simulink library "halout"  (R2021b)
settings: Solver=VariableStepAuto  StartTime=0.0  StopTime=10.0  RelTol=1e-3
undefined symbols (not defined in the file): C_TASK_5MS_S, FALSE, KHAL_CAN1FD1APS3E2E_flg, KHAL_CAN1FD1APS3TxReq_flg, KHAL_CAN1FD1VCU2E2E_flg, KHAL_CAN1FD1VCU2TxReq_flg, KHAL_CAN1FD1VCU3E2E_flg, KHAL_CAN1FD1VCU3TxReq_flg, KHAL_CAN1TxReq_flg, KHAL_CAN1VMCFCM1E2E_flg, KHAL_CAN1VMCFCM1TxReq_flg, KHAL_CAN2TxReq_flg, KHAL_CAN3FD3VCU1toNIDECTxReq_flg, KHAL_CAN3FD3VCU1TxReq_flg, KHAL_CAN3FD3VCU2E2E_flg, KHAL_CAN3FD3VCU2toNIDECE2E_flg, KHAL_CAN3FD3VCU2toNIDECTxReq_flg, KHAL_CAN3FD3VCU2TxReq_flg, KHAL_CAN3TxReq_flg, KHAL_CAN4FD4CE1000E2E_flg, KHAL_CAN4FD4CE1000TxReq_flg, KHAL_CAN4TxReq_flg, KHAL_CAN5TxReq_flg, KHAL_CAN6FD6APS3E2E_flg, KHAL_CAN6FD6APS3TxReq_flg, KHAL_CAN6FD6VCU2E2E_flg, KHAL_CAN6FD6VCU2TxReq_flg, KHAL_CAN6TxReq_flg, ONE_INT, TRUE, ZERO_INT
libraries: FVT_lib x549, simulink x244
(part 3 of 27)

== system halout/HAL_OUT/CAN1/FD1_VCU1_0x116 ==
  BSCP_outputs : Inport  OutDataTypeStr=Bus: BSCP_outputs
  BOUTP_outputs : Inport  Port=2  OutDataTypeStr=Bus: BOUTP_outputs
  CCCrlSta : Subsystem
  EngAGSCloseSta : Subsystem
  EngActvDmpDisabSta : Subsystem
  EngCoastDwSta : Subsystem
  EngPwrLockSta : Subsystem
  Ground{,1..3} (4 alike) : Ground
  HVPwrSta : Subsystem
  LVPwrSta : Subsystem
  MSACrlSta : Subsystem
  PButtonSta : Subsystem
  PrkReq : Subsystem
  PrkReqValid : Subsystem
  PwrSta : Subsystem
  ShiftGearPosn : Subsystem
  VehMalfunLevel : Subsystem
  XWDMode : Subsystem
  bus_creator : BusCreator  Inputs=15  OutDataTypeStr=Bus: DT_CAN1_SG_FD1_VCU1  NonVirtualBus=on
  bus_selector : BusSelector  OutputSignals=VOUTP_CCCtrlSta_enum
  bus_selector1 : BusSelector  OutputSignals=VOUTP_IVIPwrLockSta_enum
  bus_selector10 : BusSelector  OutputSignals=VOUTP_DrivetrainSelect_enum
  bus_selector2 : BusSelector  OutputSignals=VOUTP_HVPwrSta_flg
  bus_selector3 : BusSelector  OutputSignals=VOUTP_LVPwrSta_flg
  bus_selector4 : BusSelector  OutputSignals=VOUTP_MSACtrlSta_enum
  bus_selector5 : BusSelector  OutputSignals=VOUTP_PButtonSta_enum
  bus_selector6 : BusSelector  OutputSignals=VOUTP_ActParkRequest_flg
  bus_selector7 : BusSelector  OutputSignals=VOUTP_PowerSta_enum
  bus_selector8 : BusSelector  OutputSignals=VOUTP_ShiftGearPosn_enum
  bus_selector9 : BusSelector  OutputSignals=VOUTP_VehMalfunLevel_enum
  FD1_VCU1 : Outport
  wires:
  BSCP_outputs/1 -> [BSCP_outputs]
  BOUTP_outputs/1 -> [BOUTP_outputs]
  [CAN1_CC_Crl_Sta] -> bus_creator/1  "CAN1_CC_Crl_Sta"
  [CAN1_Eng_AGSCloseSta] -> bus_creator/2  "CAN1_Eng_AGSCloseSta"
  [CAN1_Eng_ActvDmpDisabSta] -> bus_creator/3  "CAN1_Eng_ActvDmpDisabSta"
  [CAN1_Eng_CoastDwSta] -> bus_creator/4  "CAN1_Eng_CoastDwSta"
  [CAN1_Eng_PwrLockSta] -> bus_creator/5  "CAN1_Eng_PwrLockSta"
  [CAN1_HVPwrSta] -> bus_creator/6  "CAN1_HVPwrSta"
  [CAN1_LVPwrSta] -> bus_creator/7  "CAN1_LVPwrSta"
  [CAN1_MSA_Crl_Sta] -> bus_creator/8  "CAN1_MSA_Crl_Sta"
  [CAN1_P_Button_Sta] -> bus_creator/9  "CAN1_P_Button_Sta"
  [CAN1_PrkReq] -> bus_creator/10  "CAN1_PrkReq"
  [CAN1_PrkReqValid] -> bus_creator/11  "CAN1_PrkReqValid"
  [CAN1_PwrSta] -> bus_creator/12  "CAN1_PwrSta"
  [CAN1_ShiftGearPosn] -> bus_creator/13  "CAN1_ShiftGearPosn"
  [CAN1_VehMalfunLevel] -> bus_creator/14  "CAN1_VehMalfunLevel"
  [CAN1_XWDMode] -> bus_creator/15  "CAN1_XWDMode"
  bus_creator/1 -> FD1_VCU1/1
  CCCrlSta/1(CAN1_CC_Crl_Sta) -> [CAN1_CC_Crl_Sta]
  EngAGSCloseSta/1(CAN1_Eng_AGSCloseSta) -> [CAN1_Eng_AGSCloseSta]
  EngActvDmpDisabSta/1(CAN1_Eng_ActvDmpDisabSta) -> [CAN1_Eng_ActvDmpDisabSta]
  EngCoastDwSta/1(CAN1_Eng_CoastDwSta) -> [CAN1_Eng_CoastDwSta]
  EngPwrLockSta/1(CAN1_Eng_PwrLockSta) -> [CAN1_Eng_PwrLockSta]
  HVPwrSta/1(CAN1_HVPwrSta) -> [CAN1_HVPwrSta]
  LVPwrSta/1(CAN1_LVPwrSta) -> [CAN1_LVPwrSta]
  MSACrlSta/1(CAN1_MSA_Crl_Sta) -> [CAN1_MSA_Crl_Sta]
  PButtonSta/1(CAN1_P_Button_Sta) -> [CAN1_P_Button_Sta]
  PrkReq/1(CAN1_PrkReq) -> [CAN1_PrkReq]
  PrkReqValid/1(CAN1_PrkReqValid) -> [CAN1_PrkReqValid]
  PwrSta/1(CAN1_PwrSta) -> [CAN1_PwrSta]
  ShiftGearPosn/1(CAN1_ShiftGearPosn) -> [CAN1_ShiftGearPosn]
  VehMalfunLevel/1(CAN1_VehMalfunLevel) -> [CAN1_VehMalfunLevel]
  XWDMode/1(CAN1_XWDMode) -> [CAN1_XWDMode]
  bus_selector/1 -> CCCrlSta/1(CCCrlSta)  "<VOUTP_CCCtrlSta_enum>"
  [BOUTP_outputs] -> bus_selector/1
  Ground/1 -> EngAGSCloseSta/1(EngAGSCloseSta)
  Ground1/1 -> EngActvDmpDisabSta/1(EngActvDmpDisabSta)
  Ground2/1 -> EngCoastDwSta/1(EngCoastDwSta)
  bus_selector1/1 -> EngPwrLockSta/1(EngPwrLockSta)  "<VOUTP_IVIPwrLockSta_enum>"
  [BOUTP_outputs] -> bus_selector1/1
  bus_selector2/1 -> HVPwrSta/1(HVPwrSta)  "<VOUTP_HVPwrSta_flg>"
  [BOUTP_outputs] -> bus_selector2/1
  bus_selector3/1 -> LVPwrSta/1(LVPwrSta)  "<VOUTP_LVPwrSta_flg>"
  [BOUTP_outputs] -> bus_selector3/1
  bus_selector4/1 -> MSACrlSta/1(MSACrlSta)  "<VOUTP_MSACtrlSta_enum>"
  [BOUTP_outputs] -> bus_selector4/1
  bus_selector5/1 -> PButtonSta/1(PButtonSta)  "<VOUTP_PButtonSta_enum>"
  [BOUTP_outputs] -> bus_selector5/1
  bus_selector6/1 -> PrkReq/1(PrkReq)  "<VOUTP_ActParkRequest_flg>"
  [BOUTP_outputs] -> bus_selector6/1
  Ground3/1 -> PrkReqValid/1(PrkReqValid)
  bus_selector7/1 -> PwrSta/1(PwrSta)  "<VOUTP_PowerSta_enum>"
  [BOUTP_outputs] -> bus_selector7/1
  bus_selector8/1 -> ShiftGearPosn/1(ShiftGearPosn)  "<VOUTP_ShiftGearPosn_enum>"
  [BOUTP_outputs] -> bus_selector8/1
  bus_selector9/1 -> VehMalfunLevel/1(VehMalfunLevel)  "<VOUTP_VehMalfunLevel_enum>"
  [BOUTP_outputs] -> bus_selector9/1
  bus_selector10/1 -> XWDMode/1(XWDMode)  "<VOUTP_DrivetrainSelect_enum>"
  [BOUTP_outputs] -> bus_selector10/1

== system halout/HAL_OUT/CAN1/FD1_VCU2_0x154 ==
  BSCP_outputs : Inport  OutDataTypeStr=Bus: BSCP_outputs
  BOUTP_outputs : Inport  Port=2  OutDataTypeStr=Bus: BOUTP_outputs
  Trigger : TriggerPort  TriggerType=function-call  VariantControl=(inherit)
  ACCCtrlAvail : Subsystem
  AccPedalOverride : Subsystem
  ActAPSPosn : Subsystem
  Byte_0 : Subsystem
  Byte_1 : Subsystem
  Byte_10 : Subsystem
  Byte_11 : Subsystem
  Byte_12 : Subsystem
  Byte_13 : Subsystem
  Byte_14 : Subsystem
  Byte_15 : Subsystem
  Byte_2 : Subsystem
  Byte_3 : Subsystem
  Byte_4 : Subsystem
  Byte_5 : Subsystem
  Byte_6 : Subsystem
  Byte_7 : Constant  Value=ZERO_INT
  Byte_8 : Constant  Value=ZERO_INT
  Byte_9 : Constant  Value=ZERO_INT
  CRC8_IfAction_Tx : Subsystem  AncestorBlock=FVT_lib/hal/CRC8_IfAction_Tx
      mask help: MeasumentTrigerEvent
      mask Display: fprintf('CRC8_IfAction');
  CSVCU2CAN1 : Subsystem
  Constant : Constant  Value=KHAL_CAN1FD1VCU2E2E_flg
  Constant1 : Constant  Value=0x2D
  Constant2 : Constant  Value=0xA6
  Constant3 : Constant  Value=KHAL_CAN1FD1VCU2E2E_flg
  Constant4 : Constant  Value=KHAL_CAN1FD1VCU2E2E_flg
  DriverTq : Subsystem
  FrDriverTq : Subsystem
  Ground{,1..7} (8 alike) : Ground
  Mux2 : Mux  Inputs=15
  RCVCU2CAN1 : Subsystem
  RollingCounter_IfAction : FVT_lib/hal/RollingCounter_IfAction
  RollingCounter_IfAction1 : FVT_lib/hal/RollingCounter_IfAction
  RrDriverTq : Subsystem
  Terminator : Terminator
  VehActPwr : Subsystem
  bus_creator : BusCreator  Inputs=9  OutDataTypeStr=Bus: DT_CAN1_SG_FD1_VCU2  NonVirtualBus=on
  bus_selector : BusSelector  OutputSignals=VOUTP_DriverWhlTqDemFr_Nm
  bus_selector1 : BusSelector  OutputSignals=VOUTP_DriverWhlTqDemFr_Nm
  bus_selector10 : BusSelector  OutputSignals=VOUTP_DriverWhlTqDemFr_Nm
  bus_selector11 : BusSelector  OutputSignals=VOUTP_DriverWhlTqDemRr_Nm
  bus_selector2 : BusSelector  OutputSignals=VOUTP_DriverWhlTqDemRr_Nm
  bus_selector3 : BusSelector  OutputSignals=VOUTP_DriverWhlTqDemRr_Nm
  bus_selector4 : BusSelector  OutputSignals=VOUTP_ACCCtrlAvail_flg
  bus_selector5 : BusSelector  OutputSignals=VOUTP_ACCPedalOvrd_flg
  bus_selector6 : BusSelector  OutputSignals=VOUTP_ActAPSPosn_pct
  bus_selector7 : BusSelector  OutputSignals=VOUTP_ACCCtrlAvail_flg
  bus_selector8 : BusSelector  OutputSignals=VOUTP_ACCPedalOvrd_flg
  bus_selector9 : BusSelector  OutputSignals=VOUTP_ActAPSPosn_pct
  FD1_VCU2 : Outport
  wires:
  BSCP_outputs/1 -> [BSCP_outputs]
  BOUTP_outputs/1 -> [BOUTP_outputs]
  [CAN1_ACC_CtrlAvail] -> bus_creator/1  "CAN1_ACC_CtrlAvail"
  [CAN1_AccPedal_Override] -> bus_creator/2  "CAN1_AccPedal_Override"
  [CAN1_ActAPSPosn] -> bus_creator/3  "CAN1_ActAPSPosn"
  [CAN1_CS_VCU2_CAN1] -> bus_creator/4  "CAN1_CS_VCU2_CAN1"
  [CAN1_DriverTq] -> bus_creator/5  "CAN1_DriverTq"
  [CAN1_Fr_DriverTq] -> bus_creator/6  "CAN1_Fr_DriverTq"
  [CAN1_RC_VCU2_CAN1] -> bus_creator/7  "CAN1_RC_VCU2_CAN1"
  [CAN1_Rr_DriverTq] -> bus_creator/8  "CAN1_Rr_DriverTq"
  [CAN1_VehActPwr] -> bus_creator/9  "CAN1_VehActPwr"
  bus_creator/1 -> FD1_VCU2/1
  ACCCtrlAvail/1(CAN1_ACC_CtrlAvail) -> [CAN1_ACC_CtrlAvail]
  AccPedalOverride/1(CAN1_AccPedal_Override) -> [CAN1_AccPedal_Override]
  ActAPSPosn/1(CAN1_ActAPSPosn) -> [CAN1_ActAPSPosn]
  CSVCU2CAN1/1(CAN1_CS_VCU2_CAN1) -> [CAN1_CS_VCU2_CAN1]
  DriverTq/1(CAN1_DriverTq) -> [CAN1_DriverTq]
  FrDriverTq/1(CAN1_Fr_DriverTq) -> [CAN1_Fr_DriverTq]
  RCVCU2CAN1/1(CAN1_RC_VCU2_CAN1) -> [CAN1_RC_VCU2_CAN1]
  RrDriverTq/1(CAN1_Rr_DriverTq) -> [CAN1_Rr_DriverTq]
  VehActPwr/1(CAN1_VehActPwr) -> [CAN1_VehActPwr]
  Byte_0/1(Byte_0) -> Terminator/1
  Byte_1/1(Byte_1) -> [Byte_1]
  Byte_2/1(Byte_2) -> [Byte_2]
  Byte_3/1(Byte_3) -> [Byte_3]
  Byte_4/1(Byte_4) -> [Byte_4]
  Byte_5/1(Byte_5) -> [Byte_5]
  Byte_6/1(Byte_6) -> [Byte_6]
  Byte_7/1 -> [Byte_7]
  Byte_8/1 -> [Byte_8]
  Byte_9/1 -> [Byte_9]
  Byte_10/1(Byte_10) -> [Byte_10]
  Byte_11/1(Byte_11) -> [Byte_11]
  Byte_12/1(Byte_12) -> [Byte_12]
  Byte_13/1(Byte_13) -> [Byte_13]
  Byte_14/1(Byte_14) -> [Byte_14]
  Byte_15/1(Byte_15) -> [Byte_15]
  Mux2/1 -> CRC8_IfAction_Tx/4(RawData)
  Constant/1 -> CRC8_IfAction_Tx/1(CAN_E2E_flg)
  Constant1/1 -> CRC8_IfAction_Tx/2(DataID1)
  Constant2/1 -> CRC8_IfAction_Tx/3(DataID2)
  CRC8_IfAction_Tx/1(CRC8) -> [CS_VCU2_CAN1]
  Ground/1 -> Byte_0/1(CS_VCU2_CAN1)
  [Byte_1] -> Mux2/1
  RollingCounter_IfAction/1 -> Byte_1/1(RC_VCU2_CAN1)
  Constant3/1 -> RollingCounter_IfAction/1
  [Byte_2] -> Mux2/2
  bus_selector/1 -> Byte_2/1(Fr_DriverTq)  "<VOUTP_DriverWhlTqDemFr_Nm>"
  [BOUTP_outputs] -> bus_selector/1
  [Byte_3] -> Mux2/3
  bus_selector1/1 -> Byte_3/1(Fr_DriverTq)  "<VOUTP_DriverWhlTqDemFr_Nm>"
  [BOUTP_outputs] -> bus_selector1/1
  [Byte_4] -> Mux2/4
  bus_selector2/1 -> Byte_4/1(Rr_DriverTq)  "<VOUTP_DriverWhlTqDemRr_Nm>"
  [BOUTP_outputs] -> bus_selector2/1
  [Byte_5] -> Mux2/5
  bus_selector3/1 -> Byte_5/1(Rr_DriverTq)  "<VOUTP_DriverWhlTqDemRr_Nm>"
  [BOUTP_outputs] -> bus_selector3/1
  [Byte_6] -> Mux2/6
  bus_selector4/1 -> Byte_6/1(ACC_CtrlAvail)  "<VOUTP_ACCCtrlAvail_flg>"
  [BOUTP_outputs] -> bus_selector4/1
  bus_selector5/1 -> Byte_6/2(AccPedal_Override)  "<VOUTP_ACCPedalOvrd_flg>"
  [BOUTP_outputs] -> bus_selector5/1
  [Byte_7] -> Mux2/7
  [Byte_8] -> Mux2/8
  [Byte_9] -> Mux2/9
  [Byte_10] -> Mux2/10
  Ground1/1 -> Byte_10/1(VehActPwr)
  [Byte_11] -> Mux2/11
  Ground2/1 -> Byte_11/1(VehActPwr)
  [Byte_12] -> Mux2/12
  Ground3/1 -> Byte_12/1(VehActPwr)
  [Byte_13] -> Mux2/13
  Ground4/1 -> Byte_13/1(DriverTq)
  [Byte_14] -> Mux2/14
  Ground5/1 -> Byte_14/1(DriverTq)
  [Byte_15] -> Mux2/15
  bus_selector6/1 -> Byte_15/1(ActAPSPosn)  "<VOUTP_ActAPSPosn_pct>"
  [BOUTP_outputs] -> bus_selector6/1
  bus_selector7/1 -> ACCCtrlAvail/1(ACCCtrlAvail)  "<VOUTP_ACCCtrlAvail_flg>"
  [BOUTP_outputs] -> bus_selector7/1
  bus_selector8/1 -> AccPedalOverride/1(AccPedalOverride)  "<VOUTP_ACCPedalOvrd_flg>"
  [BOUTP_outputs] -> bus_selector8/1
  bus_selector9/1 -> ActAPSPosn/1(ActAPSPosn)  "<VOUTP_ActAPSPosn_pct>"
  [BOUTP_outputs] -> bus_selector9/1
  [CS_VCU2_CAN1] -> CSVCU2CAN1/1(CSVCU2CAN1)
  Ground6/1 -> DriverTq/1(DriverTq)
  bus_selector10/1 -> FrDriverTq/1(FrDriverTq)  "<VOUTP_DriverWhlTqDemFr_Nm>"
  [BOUTP_outputs] -> bus_selector10/1
  RollingCounter_IfAction1/1 -> RCVCU2CAN1/1(RCVCU2CAN1)
  Constant4/1 -> RollingCounter_IfAction1/1
  bus_selector11/1 -> RrDriverTq/1(RrDriverTq)  "<VOUTP_DriverWhlTqDemRr_Nm>"
  [BOUTP_outputs] -> bus_selector11/1
  Ground7/1 -> VehActPwr/1(VehActPwr)

== system halout/HAL_OUT/CAN1/FD1_VCU2_Tx ==
  TxReq : Inport
  Chart : Stateflow chart  TreatAsAtomicUnit=on
  Constant : Constant  Value=C_TASK_5MS_S
  Constant3 : Constant  Value=CycleTime
  Data Type Conversion : DataTypeConversion  OutDataTypeStr=uint16
  Divide : Product  Inputs=*/
  Gain : Gain  Gain=0.001
  TxTrigger : Outport
  wires:
  Data Type Conversion/1 -> Chart/2(CycleCnt)
  Constant3/1 -> Gain/1
  Gain/1 -> Divide/1
  Chart/1(TxTrigger()) -> TxTrigger/1
  Divide/1 -> Data Type Conversion/1
  TxReq/1 -> Chart/1(TxReq)
  Constant/1 -> Divide/2

== system halout/HAL_OUT/CAN1/FD1_VCU3_0x159 ==
  BSCP_outputs : Inport  OutDataTypeStr=Bus: BSCP_outputs
  BOUTP_outputs : Inport  Port=2  OutDataTypeStr=Bus: BOUTP_outputs
  Trigger : TriggerPort  TriggerType=function-call  VariantControl=(inherit)
  Byte_0 : Subsystem
  Byte_1 : Subsystem
  Byte_10 : Subsystem
  Byte_11 : Subsystem
  Byte_12 : Subsystem
  Byte_13 : Subsystem
  Byte_14 : Subsystem
  Byte_15 : Subsystem
  Byte_16 : Subsystem
  Byte_17 : Subsystem
  Byte_18 : Subsystem
  Byte_19 : Subsystem
  Byte_2 : Constant  Value=ZERO_INT
  Byte_3 : Subsystem
  Byte_4 : Subsystem
  Byte_5 : Subsystem
  Byte_6 : Subsystem
  Byte_7 : Subsystem
  Byte_8 : Subsystem
  Byte_9 : Subsystem
  CRC8_IfAction_Tx : Subsystem  AncestorBlock=FVT_lib/hal/CRC8_IfAction_Tx
      mask help: MeasumentTrigerEvent
      mask Display: fprintf('CRC8_IfAction');
  CSVCU3CAN1 : Subsystem
  Constant : Constant  Value=KHAL_CAN1FD1VCU3E2E_flg
  Constant1 : Constant  Value=0xC8
  Constant2 : Constant  Value=0xEB
  Constant3 : Constant  Value=KHAL_CAN1FD1VCU3E2E_flg
  Constant4 : Constant  Value=KHAL_CAN1FD1VCU3E2E_flg
  EquivAccPedalSWSta : Subsystem
  FrEDUAvailBrkRgnTq : Subsystem
  FrEDUAvailBrkRgnTqValid : Subsystem
  FrEDURealARgnTq : Subsystem
  FrEDURealDrvOrBRgnTq : Subsystem
  FrEDUSpd : Subsystem
  FrEDUSpdValid : Subsystem
  FrRgnDecrSta : Subsystem
  FrRgnPermSta : Subsystem
  Ground : Ground
  Mux2 : Mux  Inputs=19
  PTCSPermSta : Subsystem
  RCVCU3CAN1 : Subsystem
  RgnAbnorSta : Subsystem
  RollingCounter_IfAction : FVT_lib/hal/RollingCounter_IfAction
  RollingCounter_IfAction1 : FVT_lib/hal/RollingCounter_IfAction
  RrEDUAvailBrkRgnTq : Subsystem
  RrEDUAvailBrkRgnTqValid : Subsystem
  RrEDURealARgnTq : Subsystem
  RrEDURealDrvOrBRgnTq : Subsystem
  RrEDUSpd : Subsystem
  RrEDUSpdValid : Subsystem
  RrRgnDecrSta : Subsystem
  RrRgnPermSta : Subsystem
  Terminator : Terminator
  bus_creator : BusCreator  Inputs=21  OutDataTypeStr=Bus: DT_CAN1_SG_FD1_VCU3  NonVirtualBus=on
  bus_selector : BusSelector  OutputSignals=VOUTP_FrEDUSpdValid_flg
  bus_selector1 : BusSelector  OutputSignals=VOUTP_FrRgnDecrSta_flg
  bus_selector10 : BusSelector  OutputSignals=VOUTP_RrEDUSpd_rpm
  bus_selector11 : BusSelector  OutputSignals=VOUTP_RrEDURolRgnTq_Nm
  bus_selector12 : BusSelector  OutputSignals=VOUTP_RrEDURolRgnTq_Nm
  bus_selector13 : BusSelector  OutputSignals=VOUTP_RrEDUAvailBrkRgnTq_Nm
  bus_selector14 : BusSelector  OutputSignals=VOUTP_RrEDUAvailBrkRgnTq_Nm
  bus_selector15 : BusSelector  OutputSignals=VOUTP_RrEDUActTq_Nm
  bus_selector16 : BusSelector  OutputSignals=VOUTP_RrEDUActTq_Nm
  bus_selector17 : BusSelector  OutputSignals=VOUTP_FrEDUAvailBrkRgnTqV_flg
  bus_selector18 : BusSelector  OutputSignals=VOUTP_FrEDUSpd_rpm
  bus_selector19 : BusSelector  OutputSignals=VOUTP_RrEDUAvailBrkRgnTqV_flg
  bus_selector2 : BusSelector  OutputSignals=VOUTP_FrRgnPermSta_flg
  bus_selector20 : BusSelector  OutputSignals=VOUTP_FrEDUSpd_rpm
  bus_selector21 : BusSelector  OutputSignals=VOUTP_FrEDURolRgnTq_Nm
  bus_selector22 : BusSelector  OutputSignals=VOUTP_FrEDURolRgnTq_Nm
  bus_selector23 : BusSelector  OutputSignals=VOUTP_FrEDUAvailBrkRgnTq_Nm
  bus_selector24 : BusSelector  OutputSignals=VOUTP_FrEDUAvailBrkRgnTq_Nm
  bus_selector25 : BusSelector  OutputSignals=VOUTP_FrEDUActTq_Nm
  bus_selector26 : BusSelector  OutputSignals=VOUTP_FrEDUActTq_Nm
  bus_selector27 : BusSelector  OutputSignals=VOUTP_EquivAccPedalSWSta_flg
  bus_selector28 : BusSelector  OutputSignals=VOUTP_FrEDUAvailBrkRgnTq_Nm
  bus_selector29 : BusSelector  OutputSignals=VOUTP_FrEDUAvailBrkRgnTqV_flg
  bus_selector3 : BusSelector  OutputSignals=VOUTP_RgnAbnorSta_flg
  bus_selector30 : BusSelector  OutputSignals=VOUTP_FrEDURolRgnTq_Nm
  bus_selector31 : BusSelector  OutputSignals=VOUTP_FrEDUActTq_Nm
  bus_selector32 : BusSelector  OutputSignals=VOUTP_FrEDUSpd_rpm
  bus_selector33 : BusSelector  OutputSignals=VOUTP_FrEDUSpdValid_flg
  bus_selector34 : BusSelector  OutputSignals=VOUTP_FrRgnDecrSta_flg
  bus_selector35 : BusSelector  OutputSignals=VOUTP_FrRgnPermSta_flg
  bus_selector36 : BusSelector  OutputSignals=VOUTP_PTCSPermSta_flg
  bus_selector37 : BusSelector  OutputSignals=VOUTP_RgnAbnorSta_flg
  bus_selector38 : BusSelector  OutputSignals=VOUTP_RrEDUAvailBrkRgnTq_Nm
  bus_selector39 : BusSelector  OutputSignals=VOUTP_RrEDUAvailBrkRgnTqV_flg
  bus_selector4 : BusSelector  OutputSignals=VOUTP_RrEDUSpdValid_flg
  bus_selector40 : BusSelector  OutputSignals=VOUTP_RrEDURolRgnTq_Nm
  bus_selector41 : BusSelector  OutputSignals=VOUTP_RrEDUActTq_Nm
  bus_selector42 : BusSelector  OutputSignals=VOUTP_RrEDUSpd_rpm
  bus_selector43 : BusSelector  OutputSignals=VOUTP_RrEDUSpdValid_flg
  bus_selector44 : BusSelector  OutputSignals=VOUTP_RrRgnDecrSta_flg
  bus_selector45 : BusSelector  OutputSignals=VOUTP_RrRgnPermSta_flg
  bus_selector5 : BusSelector  OutputSignals=VOUTP_RrRgnDecrSta_flg
  bus_selector6 : BusSelector  OutputSignals=VOUTP_RrRgnPermSta_flg
  bus_selector7 : BusSelector  OutputSignals=VOUTP_EquivAccPedalSWSta_flg
  bus_selector8 : BusSelector  OutputSignals=VOUTP_PTCSPermSta_flg
  bus_selector9 : BusSelector  OutputSignals=VOUTP_RrEDUSpd_rpm
  FD1_VCU3 : Outport
  wires:
  BSCP_outputs/1 -> [BSCP_outputs]
  BOUTP_outputs/1 -> [BOUTP_outputs]
  [CAN1_CS_VCU3_CAN1] -> bus_creator/1  "CAN1_CS_VCU3_CAN1"
  [CAN1_EquivAccPedalSWSta] -> bus_creator/2  "CAN1_EquivAccPedalSWSta"
  [CAN1_Fr_EDUAvailBrkRgnTq] -> bus_creator/3  "CAN1_Fr_EDUAvailBrkRgnTq"
  [CAN1_Fr_EDUAvailBrkRgnTqValid] -> bus_creator/4  "CAN1_Fr_EDUAvailBrkRgnTqValid"
  [CAN1_Fr_EDURealARgnTq] -> bus_creator/5  "CAN1_Fr_EDURealARgnTq"
  [CAN1_Fr_EDURealDrvOrBRgnTq] -> bus_creator/6  "CAN1_Fr_EDURealDrvOrBRgnTq"
  [CAN1_Fr_EDUSpd] -> bus_creator/7  "CAN1_Fr_EDUSpd"
  [CAN1_Fr_EDUSpdValid] -> bus_creator/8  "CAN1_Fr_EDUSpdValid"
  [CAN1_Fr_RgnDecrSta] -> bus_creator/9  "CAN1_Fr_RgnDecrSta"
  [CAN1_Fr_RgnPermSta] -> bus_creator/10  "CAN1_Fr_RgnPermSta"
  [CAN1_PTCS_PermSta] -> bus_creator/11  "CAN1_PTCS_PermSta"
  [CAN1_RC_VCU3_CAN1] -> bus_creator/12  "CAN1_RC_VCU3_CAN1"
  [CAN1_RgnAbnorSta] -> bus_creator/13  "CAN1_RgnAbnorSta"
  [CAN1_Rr_EDUAvailBrkRgnTq] -> bus_creator/14  "CAN1_Rr_EDUAvailBrkRgnTq"
  [CAN1_Rr_EDUAvailBrkRgnTqValid] -> bus_creator/15  "CAN1_Rr_EDUAvailBrkRgnTqValid"
  [CAN1_Rr_EDURealARgnTq] -> bus_creator/16  "CAN1_Rr_EDURealARgnTq"
  [CAN1_Rr_EDURealDrvOrBRgnTq] -> bus_creator/17  "CAN1_Rr_EDURealDrvOrBRgnTq"
  [CAN1_Rr_EDUSpd] -> bus_creator/18  "CAN1_Rr_EDUSpd"
  [CAN1_Rr_EDUSpdValid] -> bus_creator/19  "CAN1_Rr_EDUSpdValid"
  [CAN1_Rr_RgnDecrSta] -> bus_creator/20  "CAN1_Rr_RgnDecrSta"
  [CAN1_Rr_RgnPermSta] -> bus_creator/21  "CAN1_Rr_RgnPermSta"
  bus_creator/1 -> FD1_VCU3/1
  CSVCU3CAN1/1(CAN1_CS_VCU3_CAN1) -> [CAN1_CS_VCU3_CAN1]
  EquivAccPedalSWSta/1(CAN1_EquivAccPedalSWSta) -> [CAN1_EquivAccPedalSWSta]
  FrEDUAvailBrkRgnTq/1(CAN1_Fr_EDUAvailBrkRgnTq) -> [CAN1_Fr_EDUAvailBrkRgnTq]
  FrEDUAvailBrkRgnTqValid/1(CAN1_Fr_EDUAvailBrkRgnTqValid) -> [CAN1_Fr_EDUAvailBrkRgnTqValid]
  FrEDURealARgnTq/1(CAN1_Fr_EDURealARgnTq) -> [CAN1_Fr_EDURealARgnTq]
  FrEDURealDrvOrBRgnTq/1(CAN1_Fr_EDURealDrvOrBRgnTq) -> [CAN1_Fr_EDURealDrvOrBRgnTq]
  FrEDUSpd/1(CAN1_Fr_EDUSpd) -> [CAN1_Fr_EDUSpd]
  FrEDUSpdValid/1(CAN1_Fr_EDUSpdValid) -> [CAN1_Fr_EDUSpdValid]
  FrRgnDecrSta/1(CAN1_Fr_RgnDecrSta) -> [CAN1_Fr_RgnDecrSta]
  FrRgnPermSta/1(CAN1_Fr_RgnPermSta) -> [CAN1_Fr_RgnPermSta]
  PTCSPermSta/1(CAN1_PTCS_PermSta) -> [CAN1_PTCS_PermSta]
  RCVCU3CAN1/1(CAN1_RC_VCU3_CAN1) -> [CAN1_RC_VCU3_CAN1]
  RgnAbnorSta/1(CAN1_RgnAbnorSta) -> [CAN1_RgnAbnorSta]
  RrEDUAvailBrkRgnTq/1(CAN1_Rr_EDUAvailBrkRgnTq) -> [CAN1_Rr_EDUAvailBrkRgnTq]
  RrEDUAvailBrkRgnTqValid/1(CAN1_Rr_EDUAvailBrkRgnTqValid) -> [CAN1_Rr_EDUAvailBrkRgnTqValid]
  RrEDURealARgnTq/1(CAN1_Rr_EDURealARgnTq) -> [CAN1_Rr_EDURealARgnTq]
  RrEDURealDrvOrBRgnTq/1(CAN1_Rr_EDURealDrvOrBRgnTq) -> [CAN1_Rr_EDURealDrvOrBRgnTq]
  RrEDUSpd/1(CAN1_Rr_EDUSpd) -> [CAN1_Rr_EDUSpd]
  RrEDUSpdValid/1(CAN1_Rr_EDUSpdValid) -> [CAN1_Rr_EDUSpdValid]
  RrRgnDecrSta/1(CAN1_Rr_RgnDecrSta) -> [CAN1_Rr_RgnDecrSta]
  RrRgnPermSta/1(CAN1_Rr_RgnPermSta) -> [CAN1_Rr_RgnPermSta]
  Byte_0/1(Byte_0) -> Terminator/1
  Byte_1/1(Byte_1) -> [Byte_1]
  Byte_2/1 -> [Byte_2]
  Byte_3/1(Byte_3) -> [Byte_3]
  Byte_4/1(Byte_4) -> [Byte_4]
  Byte_5/1(Byte_5) -> [Byte_5]
  Byte_6/1(Byte_6) -> [Byte_6]
  Byte_7/1(Byte_7) -> [Byte_7]
  Byte_8/1(Byte_8) -> [Byte_8]
  Byte_9/1(Byte_9) -> [Byte_9]
  Byte_10/1(Byte_10) -> [Byte_10]
  Byte_11/1(Byte_11) -> [Byte_11]
  Byte_12/1(Byte_12) -> [Byte_12]
  Byte_13/1(Byte_13) -> [Byte_13]
  Byte_14/1(Byte_14) -> [Byte_14]
  Byte_15/1(Byte_15) -> [Byte_15]
  Byte_16/1(Byte_16) -> [Byte_16]
  Byte_17/1(Byte_17) -> [Byte_17]
  Byte_18/1(Byte_18) -> [Byte_18]
  Byte_19/1(Byte_19) -> [Byte_19]
  Mux2/1 -> CRC8_IfAction_Tx/4(RawData)
  Constant/1 -> CRC8_IfAction_Tx/1(CAN_E2E_flg)
  Constant1/1 -> CRC8_IfAction_Tx/2(DataID1)
  Constant2/1 -> CRC8_IfAction_Tx/3(DataID2)
  CRC8_IfAction_Tx/1(CRC8) -> [CS_VCU3_CAN1]
  Ground/1 -> Byte_0/1(CS_VCU3_CAN1)
  [Byte_1] -> Mux2/1
  RollingCounter_IfAction/1 -> Byte_1/1(RC_VCU3_CAN1)
  Constant3/1 -> RollingCounter_IfAction/1
  [Byte_2] -> Mux2/2
  [Byte_3] -> Mux2/3
  bus_selector/1 -> Byte_3/1(Fr_EDUSpdValid)  "<VOUTP_FrEDUSpdValid_flg>"
  [BOUTP_outputs] -> bus_selector/1
  bus_selector1/1 -> Byte_3/2(Fr_RgnDecrSta)  "<VOUTP_FrRgnDecrSta_flg>"
  [BOUTP_outputs] -> bus_selector1/1
  bus_selector2/1 -> Byte_3/3(Fr_RgnPermSta)  "<VOUTP_FrRgnPermSta_flg>"
  [BOUTP_outputs] -> bus_selector2/1
  bus_selector3/1 -> Byte_3/4(RgnAbnorSta)  "<VOUTP_RgnAbnorSta_flg>"
  [BOUTP_outputs] -> bus_selector3/1
  bus_selector4/1 -> Byte_3/5(Rr_EDUSpdValid)  "<VOUTP_RrEDUSpdValid_flg>"
  [BOUTP_outputs] -> bus_selector4/1
  bus_selector5/1 -> Byte_3/6(Rr_RgnDecrSta)  "<VOUTP_RrRgnDecrSta_flg>"
  [BOUTP_outputs] -> bus_selector5/1
  bus_selector6/1 -> Byte_3/7(Rr_RgnPermSta)  "<VOUTP_RrRgnPermSta_flg>"
  [BOUTP_outputs] -> bus_selector6/1
  [Byte_4] -> Mux2/4
  bus_selector7/1 -> Byte_4/1(EquivAccPedalSWSta)  "<VOUTP_EquivAccPedalSWSta_flg>"
  [BOUTP_outputs] -> bus_selector7/1
  bus_selector8/1 -> Byte_4/2(PTCS_PermSta)  "<VOUTP_PTCSPermSta_flg>"
  [BOUTP_outputs] -> bus_selector8/1
  bus_selector9/1 -> Byte_4/3(Rr_EDUSpd)  "<VOUTP_RrEDUSpd_rpm>"
  [BOUTP_outputs] -> bus_selector9/1
  [Byte_5] -> Mux2/5
  bus_selector10/1 -> Byte_5/1(Rr_EDUSpd)  "<VOUTP_RrEDUSpd_rpm>"
  [BOUTP_outputs] -> bus_selector10/1
  [Byte_6] -> Mux2/6
  bus_selector11/1 -> Byte_6/1(Rr_EDURealARgnTq)  "<VOUTP_RrEDURolRgnTq_Nm>"
  [BOUTP_outputs] -> bus_selector11/1
  [Byte_7] -> Mux2/7
  bus_selector12/1 -> Byte_7/1(Rr_EDURealARgnTq)  "<VOUTP_RrEDURolRgnTq_Nm>"
  [BOUTP_outputs] -> bus_selector12/1
  [Byte_8] -> Mux2/8
  bus_selector13/1 -> Byte_8/1(Rr_EDUAvailBrkRgnTq)  "<VOUTP_RrEDUAvailBrkRgnTq_Nm>"
  [BOUTP_outputs] -> bus_selector13/1
  [Byte_9] -> Mux2/9
  bus_selector14/1 -> Byte_9/1(Rr_EDUAvailBrkRgnTq)  "<VOUTP_RrEDUAvailBrkRgnTq_Nm>"
  [BOUTP_outputs] -> bus_selector14/1
  [Byte_10] -> Mux2/10
  bus_selector15/1 -> Byte_10/1(Rr_EDURealDrvOrBRgnTq)  "<VOUTP_RrEDUActTq_Nm>"
  [BOUTP_outputs] -> bus_selector15/1
  [Byte_11] -> Mux2/11
  bus_selector16/1 -> Byte_11/1(Rr_EDURealDrvOrBRgnTq)  "<VOUTP_RrEDUActTq_Nm>"
  [BOUTP_outputs] -> bus_selector16/1
  [Byte_12] -> Mux2/12
  bus_selector17/1 -> Byte_12/1(Fr_EDUAvailBrkRgnTqValid)  "<VOUTP_FrEDUAvailBrkRgnTqV_flg>"
  [BOUTP_outputs] -> bus_selector17/1
  bus_selector18/1 -> Byte_12/2(Fr_EDUSpd)  "<VOUTP_FrEDUSpd_rpm>"
  [BOUTP_outputs] -> bus_selector18/1
  bus_selector19/1 -> Byte_12/3(Rr_EDUAvailBrkRgnTqValid)  "<VOUTP_RrEDUAvailBrkRgnTqV_flg>"
  [BOUTP_outputs] -> bus_selector19/1
  [Byte_13] -> Mux2/13
  bus_selector20/1 -> Byte_13/1(Fr_EDUSpd)  "<VOUTP_FrEDUSpd_rpm>"
  [BOUTP_outputs] -> bus_selector20/1
  [Byte_14] -> Mux2/14
  bus_selector21/1 -> Byte_14/1(Fr_EDURealARgnTq)  "<VOUTP_FrEDURolRgnTq_Nm>"
  [BOUTP_outputs] -> bus_selector21/1
  [Byte_15] -> Mux2/15
  bus_selector22/1 -> Byte_15/1(Fr_EDURealARgnTq)  "<VOUTP_FrEDURolRgnTq_Nm>"
  [BOUTP_outputs] -> bus_selector22/1
  [Byte_16] -> Mux2/16
  bus_selector23/1 -> Byte_16/1(Fr_EDUAvailBrkRgnTq)  "<VOUTP_FrEDUAvailBrkRgnTq_Nm>"
  [BOUTP_outputs] -> bus_selector23/1
  [Byte_17] -> Mux2/17
  bus_selector24/1 -> Byte_17/1(Fr_EDUAvailBrkRgnTq)  "<VOUTP_FrEDUAvailBrkRgnTq_Nm>"
  [BOUTP_outputs] -> bus_selector24/1
  [Byte_18] -> Mux2/18
  bus_selector25/1 -> Byte_18/1(Fr_EDURealDrvOrBRgnTq)  "<VOUTP_FrEDUActTq_Nm>"
  [BOUTP_outputs] -> bus_selector25/1
  [Byte_19] -> Mux2/19
  bus_selector26/1 -> Byte_19/1(Fr_EDURealDrvOrBRgnTq)  "<VOUTP_FrEDUActTq_Nm>"
  [BOUTP_outputs] -> bus_selector26/1
  [CS_VCU3_CAN1] -> CSVCU3CAN1/1(CSVCU3CAN1)
  bus_selector27/1 -> EquivAccPedalSWSta/1(EquivAccPedalSWSta)  "<VOUTP_EquivAccPedalSWSta_flg>"
  [BOUTP_outputs] -> bus_selector27/1
  bus_selector28/1 -> FrEDUAvailBrkRgnTq/1(FrEDUAvailBrkRgnTq)  "<VOUTP_FrEDUAvailBrkRgnTq_Nm>"
  [BOUTP_outputs] -> bus_selector28/1
  bus_selector29/1 -> FrEDUAvailBrkRgnTqValid/1(FrEDUAvailBrkRgnTqValid)  "<VOUTP_FrEDUAvailBrkRgnTqV_flg>"
  [BOUTP_outputs] -> bus_selector29/1
  bus_selector30/1 -> FrEDURealARgnTq/1(FrEDURealARgnTq)  "<VOUTP_FrEDURolRgnTq_Nm>"
  [BOUTP_outputs] -> bus_selector30/1
  bus_selector31/1 -> FrEDURealDrvOrBRgnTq/1(FrEDURealDrvOrBRgnTq)  "<VOUTP_FrEDUActTq_Nm>"
  [BOUTP_outputs] -> bus_selector31/1
  bus_selector32/1 -> FrEDUSpd/1(FrEDUSpd)  "<VOUTP_FrEDUSpd_rpm>"
  [BOUTP_outputs] -> bus_selector32/1
  bus_selector33/1 -> FrEDUSpdValid/1(FrEDUSpdValid)  "<VOUTP_FrEDUSpdValid_flg>"
  [BOUTP_outputs] -> bus_selector33/1
  bus_selector34/1 -> FrRgnDecrSta/1(FrRgnDecrSta)  "<VOUTP_FrRgnDecrSta_flg>"
  [BOUTP_outputs] -> bus_selector34/1
  bus_selector35/1 -> FrRgnPermSta/1(FrRgnPermSta)  "<VOUTP_FrRgnPermSta_flg>"
  [BOUTP_outputs] -> bus_selector35/1
  bus_selector36/1 -> PTCSPermSta/1(PTCSPermSta)  "<VOUTP_PTCSPermSta_flg>"
  [BOUTP_outputs] -> bus_selector36/1
  RollingCounter_IfAction1/1 -> RCVCU3CAN1/1(RCVCU3CAN1)
  Constant4/1 -> RollingCounter_IfAction1/1
  bus_selector37/1 -> RgnAbnorSta/1(RgnAbnorSta)  "<VOUTP_RgnAbnorSta_flg>"
  [BOUTP_outputs] -> bus_selector37/1
  bus_selector38/1 -> RrEDUAvailBrkRgnTq/1(RrEDUAvailBrkRgnTq)  "<VOUTP_RrEDUAvailBrkRgnTq_Nm>"
  [BOUTP_outputs] -> bus_selector38/1
  bus_selector39/1 -> RrEDUAvailBrkRgnTqValid/1(RrEDUAvailBrkRgnTqValid)  "<VOUTP_RrEDUAvailBrkRgnTqV_flg>"
  [BOUTP_outputs] -> bus_selector39/1
  bus_selector40/1 -> RrEDURealARgnTq/1(RrEDURealARgnTq)  "<VOUTP_RrEDURolRgnTq_Nm>"
  [BOUTP_outputs] -> bus_selector40/1
  bus_selector41/1 -> RrEDURealDrvOrBRgnTq/1(RrEDURealDrvOrBRgnTq)  "<VOUTP_RrEDUActTq_Nm>"
  [BOUTP_outputs] -> bus_selector41/1
  bus_selector42/1 -> RrEDUSpd/1(RrEDUSpd)  "<VOUTP_RrEDUSpd_rpm>"
  [BOUTP_outputs] -> bus_selector42/1
  bus_selector43/1 -> RrEDUSpdValid/1(RrEDUSpdValid)  "<VOUTP_RrEDUSpdValid_flg>"
  [BOUTP_outputs] -> bus_selector43/1
  bus_selector44/1 -> RrRgnDecrSta/1(RrRgnDecrSta)  "<VOUTP_RrRgnDecrSta_flg>"
  [BOUTP_outputs] -> bus_selector44/1
  bus_selector45/1 -> RrRgnPermSta/1(RrRgnPermSta)  "<VOUTP_RrRgnPermSta_flg>"
  [BOUTP_outputs] -> bus_selector45/1

== system halout/HAL_OUT/CAN1/FD1_VCU3_Tx ==
  TxReq : Inport
  Chart : Stateflow chart  TreatAsAtomicUnit=on
  Constant : Constant  Value=C_TASK_5MS_S
  Constant3 : Constant  Value=CycleTime
  Data Type Conversion : DataTypeConversion  OutDataTypeStr=uint16
  Divide : Product  Inputs=*/
  Gain : Gain  Gain=0.001
  TxTrigger : Outport
  wires:
  Data Type Conversion/1 -> Chart/2(CycleCnt)
  Constant3/1 -> Gain/1
  Gain/1 -> Divide/1
  Chart/1(TxTrigger()) -> TxTrigger/1
  Divide/1 -> Data Type Conversion/1
  TxReq/1 -> Chart/1(TxReq)
  Constant/1 -> Divide/2

== system halout/HAL_OUT/CAN1/FD1_VMC1_0x17F ==
  BSCP_outputs : Inport  OutDataTypeStr=Bus: BSCP_outputs
  BOUTP_outputs : Inport  Port=2  OutDataTypeStr=Bus: BOUTP_outputs
  AccCalcuPID : Subsystem
  CCMSASpdWar : Subsystem
  DISCButtSta : Subsystem
  DISCDISCTargetSpd : Subsystem
  DISCDISCTurn : Subsystem
  DISCReqAcc : Subsystem
  DISCSta : Subsystem
  FeatArbitrFinal : Subsystem
  FeatArbitrSta : Subsystem
  FeatReqSpd : Subsystem
  FeatSetSpdFinalraw32 : Subsystem
  FrontRearSlipRatioCtrl : Subsystem
  Ground : Ground
  Ground1 : Ground
  JerkPCT : Subsystem
  LatAccCtrl : Subsystem
  LateralCtrl : Subsystem
  LimitPCT : Subsystem
  MeterIndSpeedraw32 : Subsystem
  RearWhlSlipRatioCtrl : Subsystem
  SPD2ACCAct : Subsystem
  SafetyCtrl : Subsystem
  SingleWhlSlipRatioCtrl : Subsystem
  TimeGapCalcu : Subsystem
  VMCACCCtrlAvail : Subsystem
  VMCAEBCtrlAvail : Subsystem
  VMCCCCtrlAvail : Subsystem
  VMCMSACtrlAvail : Subsystem
  VMCVCUACCCtrlAvail : Subsystem
  VMCVCUAPSCtrlAvailflg : Subsystem
  VMCVCUAccPedalOverride : Subsystem
  VMCVCUCCCrlSta : Subsystem
  VMCVCUMSACrlSta : Subsystem
  VehicleSpeedkph : Subsystem
  VehicleSpeedmph : Subsystem
  bus_creator : BusCreator  Inputs=33  OutDataTypeStr=Bus: DT_CAN1_SG_FD1_VMC1  NonVirtualBus=on
  bus_selector : BusSelector  OutputSignals=VOUTP_AccCalcuPID_mps2
  bus_selector1 : BusSelector  OutputSignals=VOUTP_CCMSASpdWar_flg
  bus_selector10 : BusSelector  OutputSignals=VOUTP_FeatSetSpdFinal_raw32
  bus_selector11 : BusSelector  OutputSignals=VOUTP_FrontRearSlipRatioCtrl_flg
  bus_selector12 : BusSelector  OutputSignals=VOUTP_JerkPCT_pct
  bus_selector13 : BusSelector  OutputSignals=VOUTP_LatAccCtrl_flg
  bus_selector14 : BusSelector  OutputSignals=VOUTP_LateralCtrl_flg
  bus_selector15 : BusSelector  OutputSignals=VOUTP_LimitPCT_pct
  bus_selector16 : BusSelector  OutputSignals=VOUTP_MeterIndSpeed_raw32
  bus_selector17 : BusSelector  OutputSignals=VOUTP_RearWhlSlipRatioCtrl_flg
  bus_selector18 : BusSelector  OutputSignals=VOUTP_SPD2ACCAct_flg
  bus_selector19 : BusSelector  OutputSignals=VOUTP_SafetyCtrl_flg
  bus_selector2 : BusSelector  OutputSignals=VOUTP_DISCReqAcc_mps2
  bus_selector20 : BusSelector  OutputSignals=VOUTP_SingleWhlSlipRatioCtrl_flg
  bus_selector21 : BusSelector  OutputSignals=VOUTP_TimeGapCalcu_s
  bus_selector22 : BusSelector  OutputSignals=VOUTP_VMCACCCtrlAvail_flg
  bus_selector23 : BusSelector  OutputSignals=VOUTP_VMCAEBCtrlAvail_flg
  bus_selector24 : BusSelector  OutputSignals=VOUTP_VMCCCCtrlAvail_flg
  bus_selector25 : BusSelector  OutputSignals=VOUTP_VMCMSACtrlAvail_flg
  bus_selector26 : BusSelector  OutputSignals=VOUTP_ACCCtrlAvail_flg
  bus_selector27 : BusSelector  OutputSignals=VOUTP_APSCtrlAvail_flg
  bus_selector28 : BusSelector  OutputSignals=VOUTP_ACCPedalOvrd_flg
  bus_selector29 : BusSelector  OutputSignals=VOUTP_CCCtrlSta_enum
  bus_selector3 : BusSelector  OutputSignals=VOUTP_DISCButtSta_flg
  bus_selector30 : BusSelector  OutputSignals=VOUTP_MSACtrlSta_enum
  bus_selector4 : BusSelector  OutputSignals=VOUTP_DISCTargetSpd_kph
  bus_selector5 : BusSelector  OutputSignals=VOUTP_DISCTurn_flg
  bus_selector6 : BusSelector  OutputSignals=VOUTP_DISCSta_enum
  bus_selector7 : BusSelector  OutputSignals=VOUTP_FeatArbitrFinal_enum
  bus_selector8 : BusSelector  OutputSignals=VOUTP_FeatArbitrSta_enum
  bus_selector9 : BusSelector  OutputSignals=VOUTP_FeatReqSpd_kph
  FD1_VMC1 : Outport
  wires:
  BSCP_outputs/1 -> [BSCP_outputs]
  BOUTP_outputs/1 -> [BOUTP_outputs]
  [CAN1_AccCalcuPID] -> bus_creator/1  "CAN1_AccCalcuPID"
  [CAN1_CCMSA_SpdWar] -> bus_creator/2  "CAN1_CCMSA_SpdWar"
  [CAN1_DISCReqAcc] -> bus_creator/3  "CAN1_DISCReqAcc"
  [CAN1_DISC_ButtSta] -> bus_creator/4  "CAN1_DISC_ButtSta"
  [CAN1_DISC_DISCTargetSpd] -> bus_creator/5  "CAN1_DISC_DISCTargetSpd"
  [CAN1_DISC_DISCTurn] -> bus_creator/6  "CAN1_DISC_DISCTurn"
  [CAN1_DISC_Sta] -> bus_creator/7  "CAN1_DISC_Sta"
  [CAN1_FeatArbitrFinal] -> bus_creator/8  "CAN1_FeatArbitrFinal"
  [CAN1_FeatArbitrSta] -> bus_creator/9  "CAN1_FeatArbitrSta"
  [CAN1_FeatReqSpd] -> bus_creator/10  "CAN1_FeatReqSpd"
  [CAN1_FeatSetSpdFinal_raw32] -> bus_creator/11  "CAN1_FeatSetSpdFinal_raw32"
  [CAN1_FrontRearSlipRatioCtrl] -> bus_creator/12  "CAN1_FrontRearSlipRatioCtrl"
  [CAN1_JerkPCT] -> bus_creator/13  "CAN1_JerkPCT"
  [CAN1_LatAccCtrl] -> bus_creator/14  "CAN1_LatAccCtrl"
  [CAN1_LateralCtrl] -> bus_creator/15  "CAN1_LateralCtrl"
  [CAN1_LimitPCT] -> bus_creator/16  "CAN1_LimitPCT"
  [CAN1_MeterIndSpeed_raw32] -> bus_creator/17  "CAN1_MeterIndSpeed_raw32"
  [CAN1_RearWhlSlipRatioCtrl] -> bus_creator/18  "CAN1_RearWhlSlipRatioCtrl"
  [CAN1_SPD2ACCAct] -> bus_creator/19  "CAN1_SPD2ACCAct"
  [CAN1_SafetyCtrl] -> bus_creator/20  "CAN1_SafetyCtrl"
  [CAN1_SingleWhlSlipRatioCtrl] -> bus_creator/21  "CAN1_SingleWhlSlipRatioCtrl"
  [CAN1_TimeGapCalcu] -> bus_creator/22  "CAN1_TimeGapCalcu"
  [CAN1_VMC_ACCCtrlAvail] -> bus_creator/23  "CAN1_VMC_ACCCtrlAvail"
  [CAN1_VMC_AEBCtrlAvail] -> bus_creator/24  "CAN1_VMC_AEBCtrlAvail"
  [CAN1_VMC_CCCtrlAvail] -> bus_creator/25  "CAN1_VMC_CCCtrlAvail"
  [CAN1_VMC_MSACtrlAvail] -> bus_creator/26  "CAN1_VMC_MSACtrlAvail"
  [CAN1_VMC_VCU_ACC_CtrlAvail] -> bus_creator/27  "CAN1_VMC_VCU_ACC_CtrlAvail"
  [CAN1_VMC_VCU_APSCtrlAvail_flg] -> bus_creator/28  "CAN1_VMC_VCU_APSCtrlAvail_flg"
  [CAN1_VMC_VCU_AccPedal_Override] -> bus_creator/29  "CAN1_VMC_VCU_AccPedal_Override"
  [CAN1_VMC_VCU_CC_Crl_Sta] -> bus_creator/30  "CAN1_VMC_VCU_CC_Crl_Sta"
  [CAN1_VMC_VCU_MSA_Crl_Sta] -> bus_creator/31  "CAN1_VMC_VCU_MSA_Crl_Sta"
  [CAN1_VehicleSpeed_kph] -> bus_creator/32  "CAN1_VehicleSpeed_kph"
  [CAN1_VehicleSpeed_mph] -> bus_creator/33  "CAN1_VehicleSpeed_mph"
  bus_creator/1 -> FD1_VMC1/1
  AccCalcuPID/1(CAN1_AccCalcuPID) -> [CAN1_AccCalcuPID]
  CCMSASpdWar/1(CAN1_CCMSA_SpdWar) -> [CAN1_CCMSA_SpdWar]
  DISCReqAcc/1(CAN1_DISCReqAcc) -> [CAN1_DISCReqAcc]
  DISCButtSta/1(CAN1_DISC_ButtSta) -> [CAN1_DISC_ButtSta]
  DISCDISCTargetSpd/1(CAN1_DISC_DISCTargetSpd) -> [CAN1_DISC_DISCTargetSpd]
  DISCDISCTurn/1(CAN1_DISC_DISCTurn) -> [CAN1_DISC_DISCTurn]
  DISCSta/1(CAN1_DISC_Sta) -> [CAN1_DISC_Sta]
  FeatArbitrFinal/1(CAN1_FeatArbitrFinal) -> [CAN1_FeatArbitrFinal]
  FeatArbitrSta/1(CAN1_FeatArbitrSta) -> [CAN1_FeatArbitrSta]
  FeatReqSpd/1(CAN1_FeatReqSpd) -> [CAN1_FeatReqSpd]
  FeatSetSpdFinalraw32/1(CAN1_FeatSetSpdFinal_raw32) -> [CAN1_FeatSetSpdFinal_raw32]
  FrontRearSlipRatioCtrl/1(CAN1_FrontRearSlipRatioCtrl) -> [CAN1_FrontRearSlipRatioCtrl]
  JerkPCT/1(CAN1_JerkPCT) -> [CAN1_JerkPCT]
  LatAccCtrl/1(CAN1_LatAccCtrl) -> [CAN1_LatAccCtrl]
  LateralCtrl/1(CAN1_LateralCtrl) -> [CAN1_LateralCtrl]
  LimitPCT/1(CAN1_LimitPCT) -> [CAN1_LimitPCT]
  MeterIndSpeedraw32/1(CAN1_MeterIndSpeed_raw32) -> [CAN1_MeterIndSpeed_raw32]
  RearWhlSlipRatioCtrl/1(CAN1_RearWhlSlipRatioCtrl) -> [CAN1_RearWhlSlipRatioCtrl]
  SPD2ACCAct/1(CAN1_SPD2ACCAct) -> [CAN1_SPD2ACCAct]
  SafetyCtrl/1(CAN1_SafetyCtrl) -> [CAN1_SafetyCtrl]
  SingleWhlSlipRatioCtrl/1(CAN1_SingleWhlSlipRatioCtrl) -> [CAN1_SingleWhlSlipRatioCtrl]
  TimeGapCalcu/1(CAN1_TimeGapCalcu) -> [CAN1_TimeGapCalcu]
  VMCACCCtrlAvail/1(CAN1_VMC_ACCCtrlAvail) -> [CAN1_VMC_ACCCtrlAvail]
  VMCAEBCtrlAvail/1(CAN1_VMC_AEBCtrlAvail) -> [CAN1_VMC_AEBCtrlAvail]
  VMCCCCtrlAvail/1(CAN1_VMC_CCCtrlAvail) -> [CAN1_VMC_CCCtrlAvail]
  VMCMSACtrlAvail/1(CAN1_VMC_MSACtrlAvail) -> [CAN1_VMC_MSACtrlAvail]
  VMCVCUACCCtrlAvail/1(CAN1_VMC_VCU_ACC_CtrlAvail) -> [CAN1_VMC_VCU_ACC_CtrlAvail]
  VMCVCUAPSCtrlAvailflg/1(CAN1_VMC_VCU_APSCtrlAvail_flg) -> [CAN1_VMC_VCU_APSCtrlAvail_flg]
  VMCVCUAccPedalOverride/1(CAN1_VMC_VCU_AccPedal_Override) -> [CAN1_VMC_VCU_AccPedal_Override]
  VMCVCUCCCrlSta/1(CAN1_VMC_VCU_CC_Crl_Sta) -> [CAN1_VMC_VCU_CC_Crl_Sta]
  VMCVCUMSACrlSta/1(CAN1_VMC_VCU_MSA_Crl_Sta) -> [CAN1_VMC_VCU_MSA_Crl_Sta]
  VehicleSpeedkph/1(CAN1_VehicleSpeed_kph) -> [CAN1_VehicleSpeed_kph]
  VehicleSpeedmph/1(CAN1_VehicleSpeed_mph) -> [CAN1_VehicleSpeed_mph]
  bus_selector/1 -> AccCalcuPID/1(AccCalcuPID)  "<VOUTP_AccCalcuPID_mps2>"
  [BOUTP_outputs] -> bus_selector/1
  bus_selector1/1 -> CCMSASpdWar/1(CCMSASpdWar)  "<VOUTP_CCMSASpdWar_flg>"
  [BOUTP_outputs] -> bus_selector1/1
  bus_selector2/1 -> DISCReqAcc/1(DISCReqAcc)  "<VOUTP_DISCReqAcc_mps2>"
  [BOUTP_outputs] -> bus_selector2/1
  bus_selector3/1 -> DISCButtSta/1(DISCButtSta)  "<VOUTP_DISCButtSta_flg>"
  [BOUTP_outputs] -> bus_selector3/1
  bus_selector4/1 -> DISCDISCTargetSpd/1(DISCDISCTargetSpd)  "<VOUTP_DISCTargetSpd_kph>"
  [BOUTP_outputs] -> bus_selector4/1
  bus_selector5/1 -> DISCDISCTurn/1(DISCDISCTurn)  "<VOUTP_DISCTurn_flg>"
  [BOUTP_outputs] -> bus_selector5/1
  bus_selector6/1 -> DISCSta/1(DISCSta)  "<VOUTP_DISCSta_enum>"
  [BOUTP_outputs] -> bus_selector6/1
  bus_selector7/1 -> FeatArbitrFinal/1(FeatArbitrFinal)  "<VOUTP_FeatArbitrFinal_enum>"
  [BOUTP_outputs] -> bus_selector7/1
  bus_selector8/1 -> FeatArbitrSta/1(FeatArbitrSta)  "<VOUTP_FeatArbitrSta_enum>"
  [BOUTP_outputs] -> bus_selector8/1
  bus_selector9/1 -> FeatReqSpd/1(FeatReqSpd)  "<VOUTP_FeatReqSpd_kph>"
  [BOUTP_outputs] -> bus_selector9/1
  bus_selector10/1 -> FeatSetSpdFinalraw32/1(FeatSetSpdFinalraw32)  "<VOUTP_FeatSetSpdFinal_raw32>"
  [BOUTP_outputs] -> bus_selector10/1
  bus_selector11/1 -> FrontRearSlipRatioCtrl/1(FrontRearSlipRatioCtrl)  "<VOUTP_FrontRearSlipRatioCtrl_flg>"
  [BOUTP_outputs] -> bus_selector11/1
  bus_selector12/1 -> JerkPCT/1(JerkPCT)  "<VOUTP_JerkPCT_pct>"
  [BOUTP_outputs] -> bus_selector12/1
  bus_selector13/1 -> LatAccCtrl/1(LatAccCtrl)  "<VOUTP_LatAccCtrl_flg>"
  [BOUTP_outputs] -> bus_selector13/1
  bus_selector14/1 -> LateralCtrl/1(LateralCtrl)  "<VOUTP_LateralCtrl_flg>"
  [BOUTP_outputs] -> bus_selector14/1
  bus_selector15/1 -> LimitPCT/1(LimitPCT)  "<VOUTP_LimitPCT_pct>"
  [BOUTP_outputs] -> bus_selector15/1
  bus_selector16/1 -> MeterIndSpeedraw32/1(MeterIndSpeedraw32)  "<VOUTP_MeterIndSpeed_raw32>"
  [BOUTP_outputs] -> bus_selector16/1
  bus_selector17/1 -> RearWhlSlipRatioCtrl/1(RearWhlSlipRatioCtrl)  "<VOUTP_RearWhlSlipRatioCtrl_flg>"
  [BOUTP_outputs] -> bus_selector17/1
  bus_selector18/1 -> SPD2ACCAct/1(SPD2ACCAct)  "<VOUTP_SPD2ACCAct_flg>"
  [BOUTP_outputs] -> bus_selector18/1
  bus_selector19/1 -> SafetyCtrl/1(SafetyCtrl)  "<VOUTP_SafetyCtrl_flg>"
  [BOUTP_outputs] -> bus_selector19/1
  bus_selector20/1 -> SingleWhlSlipRatioCtrl/1(SingleWhlSlipRatioCtrl)  "<VOUTP_SingleWhlSlipRatioCtrl_flg>"
  [BOUTP_outputs] -> bus_selector20/1
  bus_selector21/1 -> TimeGapCalcu/1(TimeGapCalcu)  "<VOUTP_TimeGapCalcu_s>"
  [BOUTP_outputs] -> bus_selector21/1
  bus_selector22/1 -> VMCACCCtrlAvail/1(VMCACCCtrlAvail)  "<VOUTP_VMCACCCtrlAvail_flg>"
  [BOUTP_outputs] -> bus_selector22/1
  bus_selector23/1 -> VMCAEBCtrlAvail/1(VMCAEBCtrlAvail)  "<VOUTP_VMCAEBCtrlAvail_flg>"
  [BOUTP_outputs] -> bus_selector23/1
  bus_selector24/1 -> VMCCCCtrlAvail/1(VMCCCCtrlAvail)  "<VOUTP_VMCCCCtrlAvail_flg>"
  [BOUTP_outputs] -> bus_selector24/1
  bus_selector25/1 -> VMCMSACtrlAvail/1(VMCMSACtrlAvail)  "<VOUTP_VMCMSACtrlAvail_flg>"
  [BOUTP_outputs] -> bus_selector25/1
  bus_selector26/1 -> VMCVCUACCCtrlAvail/1(VMCVCUACCCtrlAvail)  "<VOUTP_ACCCtrlAvail_flg>"
  [BOUTP_outputs] -> bus_selector26/1
  bus_selector27/1 -> VMCVCUAPSCtrlAvailflg/1(VMCVCUAPSCtrlAvailflg)  "<VOUTP_APSCtrlAvail_flg>"
  [BOUTP_outputs] -> bus_selector27/1
  bus_selector28/1 -> VMCVCUAccPedalOverride/1(VMCVCUAccPedalOverride)  "<VOUTP_ACCPedalOvrd_flg>"
  [BOUTP_outputs] -> bus_selector28/1
  bus_selector29/1 -> VMCVCUCCCrlSta/1(VMCVCUCCCrlSta)  "<VOUTP_CCCtrlSta_enum>"
  [BOUTP_outputs] -> bus_selector29/1
  bus_selector30/1 -> VMCVCUMSACrlSta/1(VMCVCUMSACrlSta)  "<VOUTP_MSACtrlSta_enum>"
  [BOUTP_outputs] -> bus_selector30/1
  Ground/1 -> VehicleSpeedkph/1(VehicleSpeedkph)
  Ground1/1 -> VehicleSpeedmph/1(VehicleSpeedmph)

== system halout/HAL_OUT/CAN1/FD1_VMC2_0x77 ==
  BSCP_outputs : Inport  OutDataTypeStr=Bus: BSCP_outputs
  BOUTP_outputs : Inport  Port=2  OutDataTypeStr=Bus: BOUTP_outputs
  FDCVMCRWSActvSta : Subsystem
  FDCVMCRWSDfctvSta : Subsystem
  FDCVMCRWSPositionReqCmd : Subsystem
  FDCVMCSteerFaultReqCmd : Subsystem
  Ground{,1..3} (4 alike) : Ground
  bus_creator : BusCreator  Inputs=4  OutDataTypeStr=Bus: DT_CAN1_SG_FD1_VMC2  NonVirtualBus=on
  FD1_VMC2 : Outport
  wires:
  BSCP_outputs/1 -> [BSCP_outputs]
  BOUTP_outputs/1 -> [BOUTP_outputs]
  [CAN1_FDC_VMC_RWS_Actv_Sta] -> bus_creator/1  "CAN1_FDC_VMC_RWS_Actv_Sta"
  [CAN1_FDC_VMC_RWS_Dfctv_Sta] -> bus_creator/2  "CAN1_FDC_VMC_RWS_Dfctv_Sta"
  [CAN1_FDC_VMC_RWS_PositionReq_Cmd] -> bus_creator/3  "CAN1_FDC_VMC_RWS_PositionReq_Cmd"
  [CAN1_FDC_VMC_SteerFaultReq_Cmd] -> bus_creator/4  "CAN1_FDC_VMC_SteerFaultReq_Cmd"
  bus_creator/1 -> FD1_VMC2/1
  FDCVMCRWSActvSta/1(CAN1_FDC_VMC_RWS_Actv_Sta) -> [CAN1_FDC_VMC_RWS_Actv_Sta]
  FDCVMCRWSDfctvSta/1(CAN1_FDC_VMC_RWS_Dfctv_Sta) -> [CAN1_FDC_VMC_RWS_Dfctv_Sta]
  FDCVMCRWSPositionReqCmd/1(CAN1_FDC_VMC_RWS_PositionReq_Cmd) -> [CAN1_FDC_VMC_RWS_PositionReq_Cmd]
  FDCVMCSteerFaultReqCmd/1(CAN1_FDC_VMC_SteerFaultReq_Cmd) -> [CAN1_FDC_VMC_SteerFaultReq_Cmd]
  Ground/1 -> FDCVMCRWSActvSta/1(FDCVMCRWSActvSta)
  Ground1/1 -> FDCVMCRWSDfctvSta/1(FDCVMCRWSDfctvSta)
  Ground2/1 -> FDCVMCRWSPositionReqCmd/1(FDCVMCRWSPositionReqCmd)
  Ground3/1 -> FDCVMCSteerFaultReqCmd/1(FDCVMCSteerFaultReqCmd)
